simulink model "homework2"  (R2017b)
settings: Solver=VariableStepAuto  StartTime=0.0  StopTime=10.0  RelTol=1e-3
libraries: simulink x1
settings Model: Creator=MT  LastModifiedBy=MT

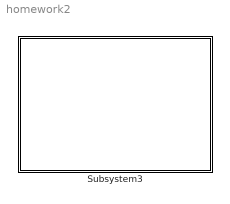
== system homework2 ==
  Subsystem3 : Subsystem

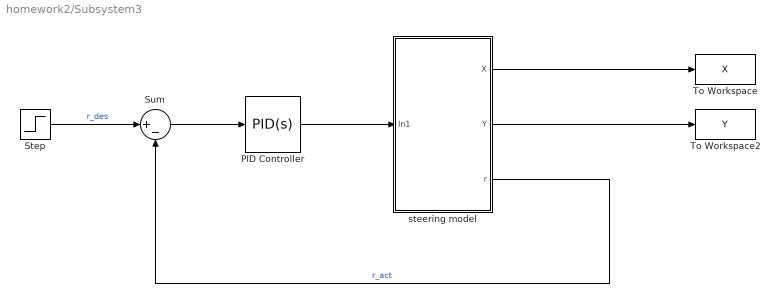
== system homework2/Subsystem3 ==
  PID Controller : simulink/Continuous/PID Controller  Controller=PID  TimeDomain=Continuous-time  SampleTime=-1  IntegratorMethod=Forward Euler  FilterMethod=Forward Euler  Form=Parallel  UseFilter=on  ControllerParametersSource=internal  P=0.261510121223526  I=1.97877056550923  D=-0.000143041548736454  N=1828.21091867052  InitialConditionSource=internal  InitialConditionForIntegrator=0  InitialConditionForFilter=0  ExternalReset=none  LimitOutput=off  UpperSaturationLimit=inf  LowerSaturationLimit=-inf  LinearizeAsGain=on  AntiWindupMode=none  Kb=1  TrackingMode=off  Kt=1  PParamMin=[]  PParamMax=[]  IParamMin=[]  IParamMax=[]  DParamMin=[]  DParamMax=[]  NParamMin=[]  NParamMax=[]  KbParamMin=[]  KbParamMax=[]  KtParamMin=[]  KtParamMax=[]  POutMin=[]  POutMax=[]  IOutMin=[]  IOutMax=[]  DOutMin=[]  DOutMax=[]  NOutMin=[]  NOutMax=[]  KbOutMin=[]  KbOutMax=[]  KtOutMin=[]  KtOutMax=[]  IntegratorOutMin=[]  IntegratorOutMax=[]  FilterOutMin=[]  FilterOutMax=[]  SumOutMin=[]  SumOutMax=[]  SumI1OutMin=[]  SumI1OutMax=[]  SumI2OutMin=[]  SumI2OutMax=[]  SumI3OutMin=[]  SumI3OutMax=[]  SumDOutMin=[]  SumDOutMax=[]  SaturationOutMin=[]  SaturationOutMax=[]  IntegratorContinuousStateAttributes=''  IntegratorStateMustResolveToSignalObject=off  IntegratorRTWStateStorageClass=Auto  FilterContinuousStateAttributes=''  FilterStateMustResolveToSignalObject=off  FilterRTWStateStorageClass=Auto  DifferentiatorICPrevScaledInput=0  DifferentiatorOutMin=[]  DifferentiatorOutMax=[]  InitialConditionSetting=State (most efficient)  FilterDiffOutCoefMin=[]  FilterDiffOutCoefMax=[]  SumDenOutMin=[]  SumDenOutMax=[]  SumNumOutMin=[]  SumNumOutMax=[]  ReciprocalOutMin=[]  ReciprocalOutMax=[]  DivideOutMin=[]  DivideOutMax=[]  TunerSelectOption=Transfer Function Based (PID Tuner App)
  Step : Step  After=23/130  SampleTime=0
  Sum : Sum  Inputs=|+-
  To Workspace : ToWorkspace  VariableName=X  SampleTime=-1
  To Workspace2 : ToWorkspace  VariableName=Y  SampleTime=-1
  steering model : Subsystem
  wires:
  PID Controller/1 -> steering model/1(In1)
  steering model/3(r) -> Sum/2  "r_act"
  steering model/2(Y) -> To Workspace2/1
  steering model/1(X) -> To Workspace/1
  Step/1 -> Sum/1  "r_des"
  Sum/1 -> PID Controller/1

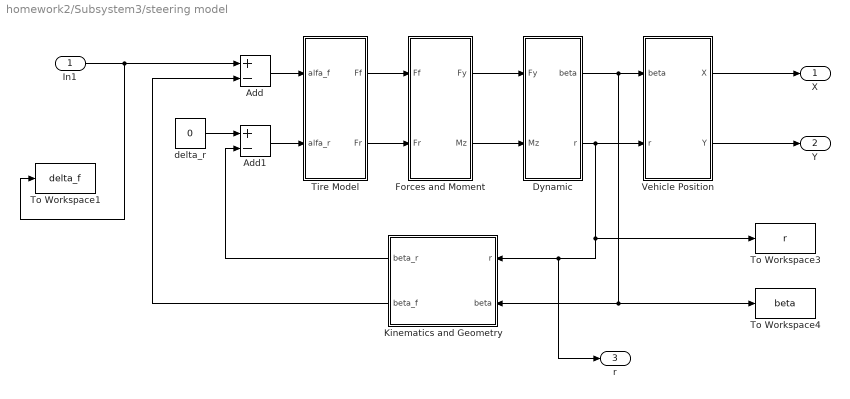
== system homework2/Subsystem3/steering model ==
  In1 : Inport
  Add : Sum  Inputs=+-
  Add1 : Sum  Inputs=+-
  Dynamic : Subsystem
  Forces and Moment : Subsystem
  Kinematics and Geometry : Subsystem
  Tire Model : Subsystem
  To Workspace1 : ToWorkspace  VariableName=delta_f  SaveFormat=Timeseries  SampleTime=-1
  To Workspace3 : ToWorkspace  VariableName=r  SaveFormat=Timeseries  SampleTime=-1
  To Workspace4 : ToWorkspace  VariableName=beta  SaveFormat=Timeseries  SampleTime=-1
  Vehicle Position : Subsystem
  delta_r : Constant  Value=0
  X : Outport
  Y : Outport  Port=2
  r : Outport  Port=3
  wires:
  Kinematics and Geometry/1(beta_r) -> Add1/2
  Dynamic/2(r) -> Vehicle Position/2(r), To Workspace3/1, r/1, Kinematics and Geometry/1(r)
  Tire Model/2(Fr) -> Forces and Moment/2(Fr)
  Tire Model/1(Ff) -> Forces and Moment/1(Ff)
  Add/1 -> Tire Model/1(alfa_f)
  delta_r/1 -> Add1/1
  In1/1 -> To Workspace1/1, Add/1
  Add1/1 -> Tire Model/2(alfa_r)
  Vehicle Position/1(X) -> X/1
  Dynamic/1(beta) -> Vehicle Position/1(beta), Kinematics and Geometry/2(beta), To Workspace4/1
  Forces and Moment/1(Fy) -> Dynamic/1(Fy)
  Forces and Moment/2(Mz) -> Dynamic/2(Mz)
  Vehicle Position/2(Y) -> Y/1
  Kinematics and Geometry/2(beta_f) -> Add/2

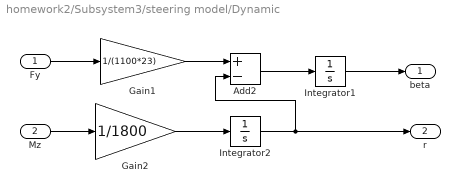
== system homework2/Subsystem3/steering model/Dynamic ==
  Fy : Inport
  Mz : Inport  Port=2
  Add2 : Sum  Inputs=+-
  Gain1 : Gain  Gain=1/(1100*23)
  Gain2 : Gain  Gain=1/1800
  Integrator1 : Integrator
  Integrator2 : Integrator
  beta : Outport
  r : Outport  Port=2
  wires:
  Fy/1 -> Gain1/1
  Integrator2/1 -> r/1, Add2/2
  Add2/1 -> Integrator1/1
  Mz/1 -> Gain2/1
  Gain2/1 -> Integrator2/1
  Integrator1/1 -> beta/1
  Gain1/1 -> Add2/1

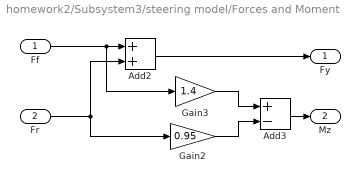
== system homework2/Subsystem3/steering model/Forces and Moment ==
  Ff : Inport
  Fr : Inport  Port=2
  Add2 : Sum
  Add3 : Sum  Inputs=+-
  Gain2 : Gain  Gain=0.95
  Gain3 : Gain  Gain=1.4
  Fy : Outport
  Mz : Outport  Port=2
  wires:
  Add2/1 -> Fy/1
  Add3/1 -> Mz/1
  Gain3/1 -> Add3/1
  Gain2/1 -> Add3/2
  Ff/1 -> Gain3/1, Add2/1
  Fr/1 -> Gain2/1, Add2/2

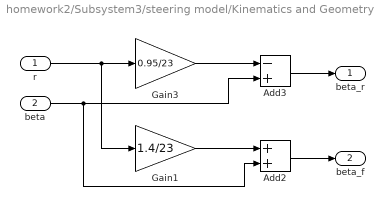
== system homework2/Subsystem3/steering model/Kinematics and Geometry ==
  r : Inport
  beta : Inport  Port=2
  Add2 : Sum
  Add3 : Sum  Inputs=-+
  Gain1 : Gain  Gain=1.4/23
  Gain3 : Gain  Gain=0.95/23
  beta_r : Outport
  beta_f : Outport  Port=2
  wires:
  Gain1/1 -> Add2/1
  beta/1 -> Add2/2, Add3/2
  Add2/1 -> beta_f/1
  Add3/1 -> beta_r/1
  r/1 -> Gain1/1, Gain3/1
  Gain3/1 -> Add3/1

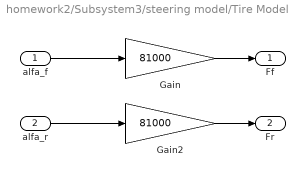
== system homework2/Subsystem3/steering model/Tire Model ==
  alfa_f : Inport
  alfa_r : Inport  Port=2
  Gain : Gain  Gain=81000
  Gain2 : Gain  Gain=81000
  Ff : Outport
  Fr : Outport  Port=2
  wires:
  Gain2/1 -> Fr/1
  alfa_r/1 -> Gain2/1
  Gain/1 -> Ff/1
  alfa_f/1 -> Gain/1

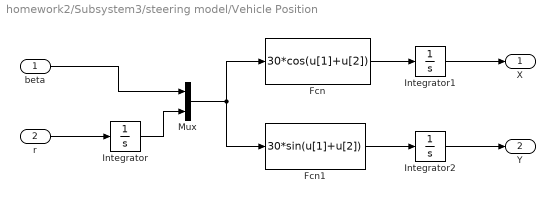
== system homework2/Subsystem3/steering model/Vehicle Position ==
  beta : Inport
  r : Inport  Port=2
  Fcn : Fcn  Expr=30*cos(u[1]+u[2])
  Fcn1 : Fcn  Expr=30*sin(u[1]+u[2])
  Integrator : Integrator
  Integrator1 : Integrator
  Integrator2 : Integrator
  Mux : Mux  Inputs=2
  X : Outport
  Y : Outport  Port=2
  wires:
  Integrator1/1 -> X/1
  Integrator2/1 -> Y/1
  Fcn/1 -> Integrator1/1
  Integrator/1 -> Mux/2
  Mux/1 -> Fcn1/1, Fcn/1
  r/1 -> Integrator/1
  beta/1 -> Mux/1
  Fcn1/1 -> Integrator2/1
